simulink model "fxpdemo_interp_precision"  (Simulink 7.6)
settings: Solver=FixedStepDiscrete  StartTime=0.0  StopTime=10.0  FixedStep=1  RelTol=1e-3
Description:
  | High Precision Calculations in Interpolation Block
  | The Interpolation Using Prelookup block allows the data type for intermediate results to be set.
  | 
  | In this model, the table is stored using an 8-bit data type, and the calculations are performed
  | using a 16-bit data type. The default *Intermediate results data type* is |Inherit: Inherit via
  | internal rule| that tries to maximize the precision of the intermediate results.
  | 
  | To see this in the generated code, open the model and build it.
settings Model: Creator=The MathWorks Inc.
settings DataIOCC: SaveFormat=StructureWithTime
settings OptimizationCC: InlineParams=on
settings DebuggingCC: ParameterPrecisionLossMsg=none  StrictBusMsg=Warning
settings RTWCC: GenCodeOnly=on  GenerateReport=on  RTWVerbose=off  ProcessScript=grt_make_rtw_hook  LaunchReport=on

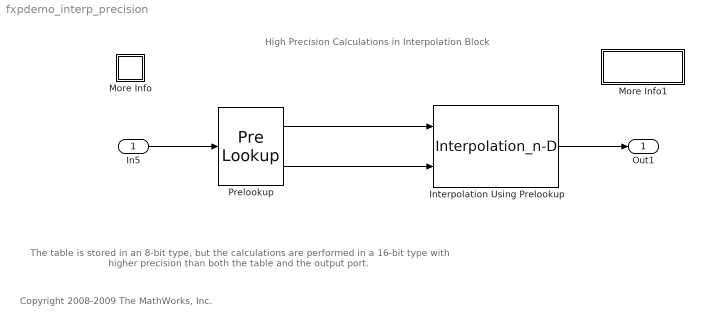
== system fxpdemo_interp_precision ==
  note: Copyright 2008-2009 The MathWorks, Inc.
  note: The table is stored in an 8-bit type, but the calculations are performed
      | in a 16-bit type with higher precision than both the table and the output port.
  note: High Precision Calculations in Interpolation Block
  In5 : Inport  OutDataTypeStr=fixdt(1,16,2^-5,0)
  Interpolation Using Prelookup : Interpolation_n-D  NumberOfTableDimensions=1  Table=sin(linspace(0,pi/4,11))  ExtrapMethod=None - Clip  CheckIndexInCode=off  OutDataTypeStr=fixdt(1,16,2^-8,0)  TableDataTypeStr=fixdt(0,8,8)  IntermediateResultsDataTypeStr=fixdt(0,16,16)
      settings: AttributesFormatString=Table type = %<TableDataTypeStr>\nIntermediate type = %<IntermediateResultsDataTypeStr>  InputPortMap=u0,u1
  More Info : Subsystem
      settings: OpenFcn=showdemo(bdroot(gcs))
      mask Display: disp('?')
  More Info1 : Subsystem
      settings: OpenFcn=rtwbuild(bdroot(gcs))
      mask Display: fprintf('Double-click to\ngenerate code')
  Prelookup : PreLookup  BreakpointsData=exp(linspace(1,3,11))  BreakpointDataTypeStr=fixdt(1,16,10)  FractionDataTypeStr=fixdt(1,16,14)
  Out1 : Outport
  wires:
  Interpolation Using Prelookup/1 -> Out1/1
  In5/1 -> Prelookup/1
  Prelookup/1 -> Interpolation Using Prelookup/1
  Prelookup/2 -> Interpolation Using Prelookup/2

== system fxpdemo_interp_precision/More Info ==

== system fxpdemo_interp_precision/More Info1 ==
